simulink model "test_loopback_mux"  (Simulink 7.0)
settings: Solver=ode45  StartTime=0.0  StopTime=4000  RelTol=1e-3
libraries: xbsIndex_r4 x498, xps_library x21, xbsReplacements_r4 x18, casper_library x15
(part 1 of 3)
settings Model: Creator=dsp  LastModifiedBy=dsp
settings DebuggingCC: SaveWithParameterizedLinksMsg=none  SignalResolutionControl=TryResolveAllWithWarning  MultiTaskDSMMsg=warning  MultiTaskCondExecSysMsg=none  StrictBusMsg=None
settings RTWCC: IncludeERTFirstTime=on
settings GRTTargetCC: TargetFcnLib=ansi_tfl_tmw.mat

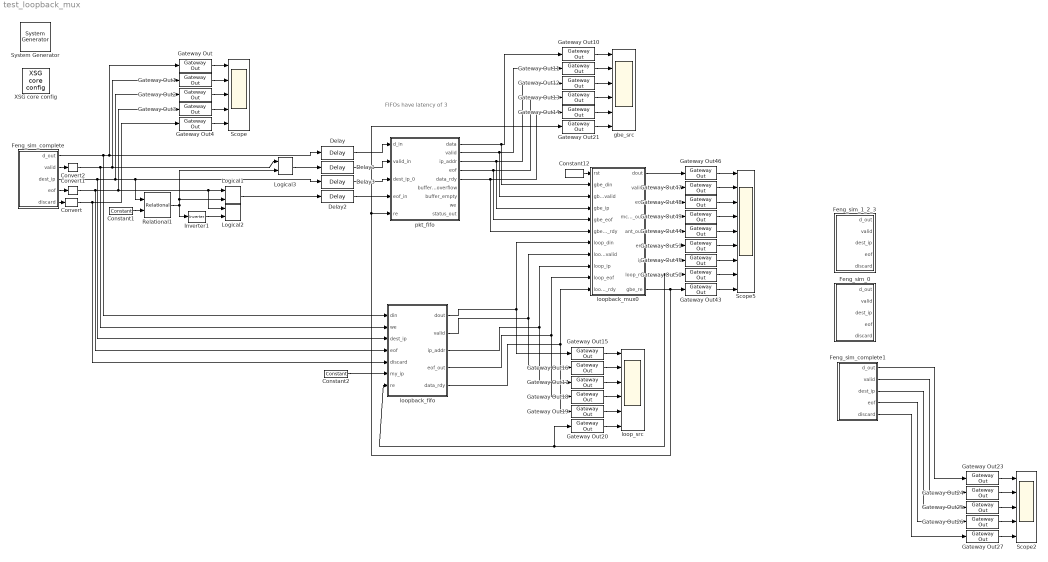
== system test_loopback_mux ==
  note: FIFOs have latency of 3
  " System Generator" : xbsIndex_r4/ System Generator  Tag=genX  SystemSampleTime=-1  xilinxfamily=Virtex2P  part=xc2vp70  speed=-7  package=ff1704  synthesis_tool=XST  clock_wrapper=Clock Enables  directory=./b_2x_8a_r308d/sysgen  testbench=off  simulink_period=1  sysclk_period=4.878  dcm_input_clock_period=100  incr_netlist=off  trim_vbits=Everywhere in SubSystem  dbl_ovrd=According to Block Masks  core_generation=According to Block Masks  run_coregen=off  deprecated_control=off  eval_field=0  block_type=sysgen
      settings: block_version=10.1.3
  Constant1 : xbsIndex_r4/Constant  arith_type=Unsigned  const=0  n_bits=1  bin_pt=0  explicit_period=on  period=1  equ=P=C  opselect=C  inp2=PCIN>>17  opr=+  inp1=P  carry=CIN  dbl_ovrd=off  block_type=constant
  Constant12 : xbsIndex_r4/Constant  arith_type=Boolean  const=0  n_bits=1  bin_pt=0  explicit_period=on  period=1  equ=P=C  opselect=C  inp2=PCIN>>17  opr=+  inp1=P  carry=CIN  dbl_ovrd=off  block_type=constant
  Constant2 : xbsIndex_r4/Constant  arith_type=Unsigned  const=0  n_bits=32  bin_pt=0  explicit_period=on  period=1  equ=P=C  opselect=C  inp2=PCIN>>17  opr=+  inp1=P  carry=CIN  dbl_ovrd=off  block_type=constant
  Convert : xbsIndex_r4/Convert  arith_type=Boolean  n_bits=8  bin_pt=6  quantization=Truncate  overflow=Wrap  latency=0  dbl_ovrd=off  pipeline=off  block_type=convert
      settings: xl_area=[0, 0, 0, 0, 0, 0, 0]  block_version=10.1.3
  Convert1 : xbsIndex_r4/Convert  arith_type=Boolean  n_bits=8  bin_pt=6  quantization=Truncate  overflow=Wrap  latency=0  dbl_ovrd=off  pipeline=off  block_type=convert
      settings: xl_area=[0, 0, 0, 0, 0, 0, 0]  block_version=10.1.3
  Convert2 : xbsIndex_r4/Convert  arith_type=Boolean  n_bits=8  bin_pt=6  quantization=Truncate  overflow=Wrap  latency=0  dbl_ovrd=off  pipeline=off  block_type=convert
      settings: xl_area=[0, 0, 0, 0, 0, 0, 0]  block_version=10.1.3
  Delay{,1..3} (4 alike) : xbsIndex_r4/Delay  en=off  latency=220  dbl_ovrd=off  reg_retiming=off  block_type=delay
      settings: xl_area=[0, 0, 0, 0, 0, 0, 0]
  Feng_sim_0 : Subsystem
  Feng_sim_1_2_3 : Subsystem
  Feng_sim_complete : Subsystem
  Feng_sim_complete1 : Subsystem
  Gateway Out{,1..4,10..21,23..27,43..51} (31 alike) : xbsIndex_r4/Gateway Out  hdl_port=on  timing_constraint=None  locs_specified=off  LOCs={}  block_type=gatewayout
      settings: infoedit="Gateway out block.  Converts Xilinx fixed point inputs into ouputs of type Simulink integer, double, or fixed point.<P><P>Hardware notes:  In hardware these blocks become top level output ports or are discarded, depending on how they are configured."  xl_area=[0, 0, 0, 0, 0, 0, 0]  block_version=10.1.3
  Inverter1 : xbsIndex_r4/Inverter  en=off  latency=0  dbl_ovrd=off  block_type=inv
      settings: xl_area=[0, 0, 0, 0, 0, 0, 0]
  Logical1 : xbsIndex_r4/Logical  logical_function=AND  inputs=2  en=off  latency=0  precision=Full  arith_type=Unsigned  n_bits=8  bin_pt=2  align_bp=on  dbl_ovrd=off  block_type=logical
      settings: xl_area=[0, 0, 0, 0, 0, 0, 0]
  Logical2 : xbsIndex_r4/Logical  logical_function=AND  inputs=2  en=off  latency=0  precision=Full  arith_type=Unsigned  n_bits=8  bin_pt=2  align_bp=on  dbl_ovrd=off  block_type=logical
      settings: xl_area=[0, 0, 0, 0, 0, 0, 0]
  Logical3 : xbsIndex_r4/Logical  logical_function=AND  inputs=2  en=off  latency=0  precision=Full  arith_type=Unsigned  n_bits=8  bin_pt=2  align_bp=on  dbl_ovrd=off  block_type=logical
      settings: xl_area=[0, 0, 0, 0, 0, 0, 0]
  Relational1 : xbsIndex_r4/Relational  mode=a!=b  en=off  latency=0  dbl_ovrd=off  block_type=relational
      settings: xl_area=[0, 0, 0, 0, 0, 0, 0]  block_version=10.1.3
  Scope : Scope  NumInputPorts=5
      settings: TimeRange=10000  YMin=0~0~0~0~-1  YMax=5000~1~3~1~1
  Scope2 : Scope  NumInputPorts=5
      settings: TimeRange=10000  YMin=0~0~0~0~-1  YMax=5000~1~3~1~1  SaveName=ScopeData12
  Scope5 : Scope  NumInputPorts=9
      settings: YMin=1100~0~0~-1~0.95~-5~-5~-5~-5  YMax=1200~1~1~1~1.05~5~5~5~5  SaveName=ScopeData17
  XSG core config : xps_library/XSG core config  Tag=xps:xsg  SystemSampleTime=-1  hw_sys=BEE2_usr  ibob_linux=off  clk_src=sys_clk  iBOB_clk_src=sys_clk  BEE2_ctrl_clk_src=sys_clk  BEE2_usr_clk_src=sys_clk  ROACH_clk_src=sys_clk  CORR_clk_src=sys_clk  gpio_clk_io_group=iBOB:sma  gpio_clk_bit_index=0  clk_rate=100  sample_period=1  synthesis_tool=XST  mpc_type=powerpc405
  gbe_src : Scope  NumInputPorts=6
      settings: YMin=95.95~0.95~1.9~-1~-1~-1  YMax=106.05~1.05~2.1~1~1~1  SaveName=ScopeData4
  loop_src : Scope  NumInputPorts=6
      settings: YMin=95.95~0.95~1.9~-1~-1~-1  YMax=106.05~1.05~2.1~1~1~1
  loopback_fifo : Subsystem
  loopback_mux0 : Subsystem  mask{timeout_bits=12, payload_len=50, fifo_latency=3}
      mask prompts: timeout_bits "Timeout (clock cycles, 2^?)"; payload_len "Expected payload length (in 64bit words)"; fifo_latency "Input pkt_fifo latencies"
      mask init:
      | payload_bits = ceil(log2(payload_len));
      | fmtstr = sprintf('Payload Len: %i\nFIFO latencies: %i.', payload_len,fifo_latency);
      | set_param(gcb, 'AttributesFormatString', fmtstr);
      settings: AttributesFormatString=|
      | Payload Len: 50
      | FIFO latencies: 3.
  pkt_fifo : Subsystem
      settings: AttributesFormatString=|
      | Max 1024 data words.
      | Max 32 pkts.
  wires:
  Feng_sim_complete/1(d_out) -> Gateway Out/1, Delay/1, loopback_fifo/1(din)
  Feng_sim_complete/2(valid) -> Convert2/1
  Feng_sim_complete/4(eof) -> Convert1/1
  Feng_sim_complete/3(dest_ip) -> Gateway Out2/1, Relational1/1, Delay3/1, loopback_fifo/3(dest_ip)
  Feng_sim_complete/5(discard) -> Convert/1
  Gateway Out/1 -> Scope/1
  Gateway Out1/1 -> Scope/2
  Gateway Out2/1 -> Scope/3
  Gateway Out3/1 -> Scope/4
  Gateway Out4/1 -> Scope/5
  Inverter1/1 -> Logical2/2
  Relational1/1 -> Inverter1/1, Logical1/2, Logical3/2
  Logical1/1 -> Delay2/1
  Constant1/1 -> Relational1/2
  Gateway Out10/1 -> gbe_src/1
  Gateway Out11/1 -> gbe_src/2
  Gateway Out12/1 -> gbe_src/3
  Gateway Out13/1 -> gbe_src/4
  Gateway Out14/1 -> gbe_src/5
  Gateway Out21/1 -> gbe_src/6
  Feng_sim_complete1/1(d_out) -> Gateway Out23/1
  Feng_sim_complete1/2(valid) -> Gateway Out24/1
  Feng_sim_complete1/3(dest_ip) -> Gateway Out25/1
  Feng_sim_complete1/4(eof) -> Gateway Out26/1
  Feng_sim_complete1/5(discard) -> Gateway Out27/1
  Gateway Out23/1 -> Scope2/1
  Gateway Out24/1 -> Scope2/2
  Gateway Out25/1 -> Scope2/3
  Gateway Out26/1 -> Scope2/4
  Gateway Out27/1 -> Scope2/5
  Gateway Out46/1 -> Scope5/1
  Gateway Out47/1 -> Scope5/2
  Gateway Out48/1 -> Scope5/3
  Gateway Out49/1 -> Scope5/4
  Gateway Out44/1 -> Scope5/5
  pkt_fifo/1(data) -> Gateway Out10/1, loopback_mux0/2(gbe_din)
  pkt_fifo/2(valid) -> Gateway Out11/1, loopback_mux0/3(gbe_valid)
  pkt_fifo/3(ip_addr) -> Gateway Out12/1, loopback_mux0/4(gbe_ip)
  Gateway Out15/1 -> loop_src/1
  Gateway Out16/1 -> loop_src/2
  Gateway Out17/1 -> loop_src/3
  Gateway Out18/1 -> loop_src/4
  Gateway Out19/1 -> loop_src/5
  Gateway Out20/1 -> loop_src/6
  Gateway Out51/1 -> Scope5/6
  Gateway Out45/1 -> Scope5/7
  Gateway Out50/1 -> Scope5/8
  Gateway Out43/1 -> Scope5/9
  loopback_mux0/1(dout) -> Gateway Out46/1
  loopback_mux0/2(valid) -> Gateway Out47/1
  loopback_mux0/3(eof) -> Gateway Out48/1
  loopback_mux0/4(mcnt_out) -> Gateway Out49/1
  loopback_mux0/5(ant_out) -> Gateway Out44/1
  loopback_mux0/6(err) -> Gateway Out51/1
  loopback_mux0/7(ip) -> Gateway Out45/1
  loopback_mux0/8(loop_re) -> Gateway Out50/1, Gateway Out20/1, loopback_fifo/7(re)
  loopback_mux0/9(gbe_re) -> Gateway Out43/1, pkt_fifo/5(re), Gateway Out21/1
  Logical3/1 -> Delay1/1
  Delay/1 -> pkt_fifo/1(d_in)
  Delay1/1 -> pkt_fifo/2(valid_in)
  Delay3/1 -> pkt_fifo/3(dest_ip_0)
  Delay2/1 -> pkt_fifo/4(eof_in)
  pkt_fifo/4(eof) -> Gateway Out13/1, loopback_mux0/5(gbe_eof)
  Constant12/1 -> loopback_mux0/1(rst)
  loopback_fifo/1(dout) -> loopback_mux0/7(loop_din), Gateway Out15/1
  loopback_fifo/2(valid) -> loopback_mux0/8(loop_valid), Gateway Out16/1
  loopback_fifo/3(ip_addr) -> loopback_mux0/9(loop_ip), Gateway Out17/1
  pkt_fifo/5(data_rdy) -> Gateway Out14/1, loopback_mux0/6(gbe_data_rdy)
  loopback_fifo/5(data_rdy) -> loopback_mux0/11(loop_data_rdy), Gateway Out19/1
  Convert/1 -> Gateway Out4/1, loopback_fifo/5(discard)
  Convert1/1 -> Gateway Out3/1, Logical1/1, Logical2/1, loopback_fifo/4(eof)
  Convert2/1 -> Gateway Out1/1, Logical3/1, loopback_fifo/2(we)
  Constant2/1 -> loopback_fifo/6(my_ip)
  loopback_fifo/4(eof_out) -> loopback_mux0/10(loop_eof), Gateway Out18/1

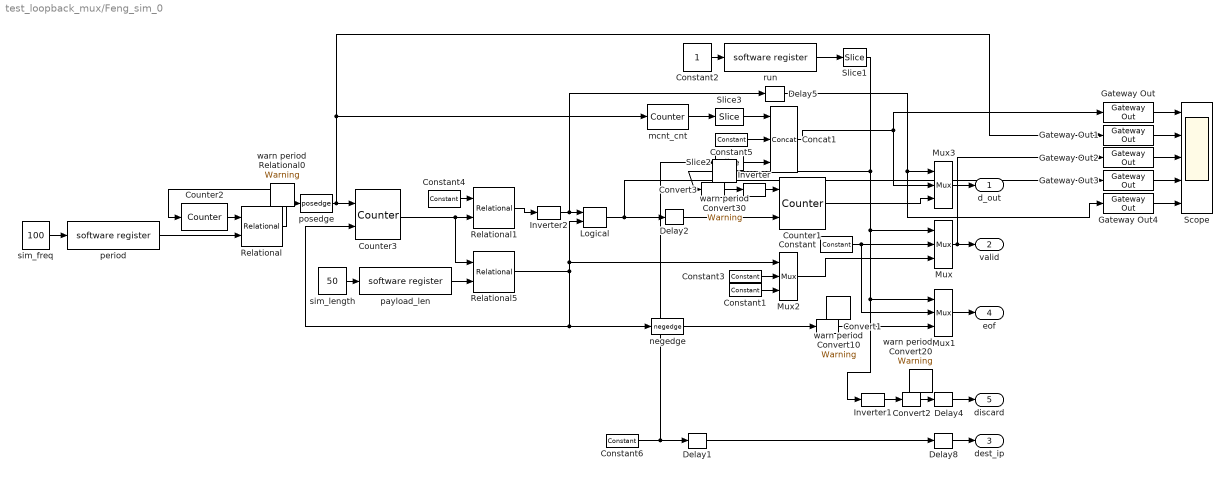
== system test_loopback_mux/Feng_sim_0 ==
  Concat1 : xbsIndex_r4/Concat  num_inputs=3  dbl_ovrd=off  block_type=concat
      settings: block_version=10.1.3
  Constant : xbsIndex_r4/Constant  arith_type=Boolean  const=0  n_bits=1  bin_pt=0  explicit_period=on  period=1  equ=P=C  opselect=C  inp2=PCIN>>17  opr=+  inp1=P  carry=CIN  dbl_ovrd=off  block_type=constant
  Constant1 : xbsIndex_r4/Constant  arith_type=Boolean  const=1  n_bits=1  bin_pt=0  explicit_period=off  period=1  equ=P=C  opselect=C  inp2=PCIN>>17  opr=+  inp1=P  carry=CIN  dbl_ovrd=off  block_type=constant
  Constant2 : Constant  OutDataType=sfix(16)  OutScaling=2^0
  Constant3 : xbsIndex_r4/Constant  arith_type=Boolean  const=0  n_bits=1  bin_pt=0  explicit_period=off  period=1  equ=P=C  opselect=C  inp2=PCIN>>17  opr=+  inp1=P  carry=CIN  dbl_ovrd=off  block_type=constant
  Constant4 : xbsIndex_r4/Constant  arith_type=Unsigned  const=0  n_bits=32  bin_pt=0  explicit_period=on  period=1  equ=P=C  opselect=C  inp2=PCIN>>17  opr=+  inp1=P  carry=CIN  dbl_ovrd=off  block_type=constant
  Constant5 : xbsIndex_r4/Constant  arith_type=Unsigned  const=0  n_bits=16-2  bin_pt=0  explicit_period=on  period=1  equ=P=C  opselect=C  inp2=PCIN>>17  opr=+  inp1=P  carry=CIN  dbl_ovrd=off  block_type=constant
  Constant6 : xbsIndex_r4/Constant  arith_type=Unsigned  const=0  n_bits=32  bin_pt=0  explicit_period=on  period=1  equ=P=C  opselect=C  inp2=PCIN>>17  opr=+  inp1=P  carry=CIN  dbl_ovrd=off  block_type=constant
  Convert1 : xbsIndex_r4/Convert  arith_type=Boolean  n_bits=8  bin_pt=6  quantization=Truncate  overflow=Wrap  latency=0  dbl_ovrd=off  pipeline=off  block_type=convert
      settings: xl_area=[0, 0, 0, 0, 0, 0, 0]  block_version=10.1.3
  Convert2 : xbsIndex_r4/Convert  arith_type=Boolean  n_bits=8  bin_pt=6  quantization=Truncate  overflow=Wrap  latency=0  dbl_ovrd=off  pipeline=off  block_type=convert
      settings: xl_area=[0, 0, 0, 0, 0, 0, 0]  block_version=10.1.3
  Convert3 : xbsIndex_r4/Convert  arith_type=Boolean  n_bits=8  bin_pt=6  quantization=Truncate  overflow=Wrap  latency=0  dbl_ovrd=off  pipeline=off  block_type=convert
      settings: xl_area=[0, 0, 0, 0, 0, 0, 0]  block_version=10.1.3
  Counter1 : xbsIndex_r4/Counter  cnt_type=Free Running  cnt_to=Inf  operation=Up  start_count=0  cnt_by_val=1  arith_type=Unsigned  n_bits=64  bin_pt=0  load_pin=off  rst=on  en=on  explicit_period=off  period=1  dbl_ovrd=off  use_behavioral_HDL=off  use_rpm=off  implementation=Fabric  block_type=counter
      settings: xl_area=[0, 0, 0, 0, 0, 0, 0]
  Counter2 : xbsIndex_r4/Counter  cnt_type=Free Running  cnt_to=Inf  operation=Up  start_count=1  cnt_by_val=1  arith_type=Unsigned  n_bits=32  bin_pt=0  load_pin=off  rst=on  en=off  explicit_period=on  period=1  dbl_ovrd=off  use_behavioral_HDL=off  use_rpm=on  implementation=Fabric  block_type=counter
      settings: xl_area=[0, 0, 0, 0, 0, 0, 0]
  Counter3 : xbsIndex_r4/Counter  cnt_type=Free Running  cnt_to=1023  operation=Up  start_count=0  cnt_by_val=1  arith_type=Unsigned  n_bits=32  bin_pt=0  load_pin=off  rst=on  en=on  explicit_period=on  period=1  dbl_ovrd=off  use_behavioral_HDL=off  use_rpm=on  implementation=Fabric  block_type=counter
      settings: xl_area=[0, 0, 0, 0, 0, 0, 0]
  Delay{1..2,4..5,8} (5 alike) : xbsIndex_r4/Delay  en=off  latency=1  dbl_ovrd=off  reg_retiming=on  block_type=delay
      settings: xl_area=[0, 0, 0, 0, 0, 0, 0]
  Gateway Out{,1..4} (5 alike) : xbsIndex_r4/Gateway Out  hdl_port=on  timing_constraint=None  locs_specified=off  LOCs={}  block_type=gatewayout
      settings: infoedit="Gateway out block.  Converts Xilinx fixed point inputs into ouputs of type Simulink integer, double, or fixed point.<P><P>Hardware notes:  In hardware these blocks become top level output ports or are discarded, depending on how they are configured."  xl_area=[0, 0, 0, 0, 0, 0, 0]  block_version=10.1.3
  Inverter : xbsIndex_r4/Inverter  en=off  latency=0  dbl_ovrd=off  block_type=inv
      settings: xl_area=[0, 0, 0, 0, 0, 0, 0]
  Inverter1 : xbsIndex_r4/Inverter  en=off  latency=0  dbl_ovrd=off  block_type=inv
      settings: xl_area=[0, 0, 0, 0, 0, 0, 0]
  Inverter2 : xbsIndex_r4/Inverter  en=off  latency=0  dbl_ovrd=off  block_type=inv
      settings: xl_area=[0, 0, 0, 0, 0, 0, 0]
  Logical : xbsIndex_r4/Logical  logical_function=AND  inputs=2  en=off  latency=0  precision=Full  arith_type=Unsigned  n_bits=8  bin_pt=2  align_bp=on  dbl_ovrd=off  block_type=logical
      settings: xl_area=[0, 0, 0, 0, 0, 0, 0]
  Mux{,1..3} (4 alike) : xbsIndex_r4/Mux  inputs=2  en=off  latency=1  precision=Full  arith_type="Signed  (2's comp)"  n_bits=8  bin_pt=2  quantization=Truncate  overflow=Wrap  dbl_ovrd=off  block_type=mux
      settings: xl_area=[0, 0, 0, 0, 0, 0, 0]
  Relational : xbsIndex_r4/Relational  mode=a>=b  en=off  latency=0  dbl_ovrd=off  block_type=relational
      settings: xl_area=[0, 0, 0, 0, 0, 0, 0]  block_version=10.1.3
  Relational1 : xbsIndex_r4/Relational  mode=a=b  en=off  latency=0  dbl_ovrd=off  block_type=relational
      settings: xl_area=[0, 0, 0, 0, 0, 0, 0]  block_version=10.1.3
  Relational5 : xbsIndex_r4/Relational  mode=a<=b  en=off  latency=0  dbl_ovrd=off  block_type=relational
      settings: xl_area=[0, 0, 0, 0, 0, 0, 0]  block_version=10.1.3
  Scope : Scope  NumInputPorts=5
      settings: TimeRange=4000  YMin=130000~0~0~0~0  YMax=200000~1~1~1~1  SaveName=ScopeData11
  Slice1 : xbsIndex_r4/Slice  nbits=1  boolean_output=off  mode=Lower Bit Location + Width  bit1=1  base1=MSB of Input  bit0=0  base0=LSB of Input  dbl_ovrd=off  block_type=slice
      settings: infoedit="Extracts a given range of bits from each input sample and presents it at the output.  The output type is ordinarily unsigned with binary point at zero, but can be Boolean when the slice is one bit wide.<P><P>Hardware notes: In hardware this block costs nothing."  block_version=10.1.3
  Slice2 : xbsIndex_r4/Slice  nbits=2  boolean_output=off  mode=Lower Bit Location + Width  bit1=1  base1=MSB of Input  bit0=0  base0=LSB of Input  dbl_ovrd=off  block_type=slice
      settings: infoedit="Extracts a given range of bits from each input sample and presents it at the output.  The output type is ordinarily unsigned with binary point at zero, but can be Boolean when the slice is one bit wide.<P><P>Hardware notes: In hardware this block costs nothing."  block_version=10.1.3
  Slice3 : xbsIndex_r4/Slice  nbits=48  boolean_output=off  mode=Lower Bit Location + Width  bit1=1  base1=MSB of Input  bit0=2  base0=LSB of Input  dbl_ovrd=off  block_type=slice
      settings: infoedit="Extracts a given range of bits from each input sample and presents it at the output.  The output type is ordinarily unsigned with binary point at zero, but can be Boolean when the slice is one bit wide.<P><P>Hardware notes: In hardware this block costs nothing."  block_version=10.1.3
  mcnt_cnt : xbsIndex_r4/Counter  cnt_type=Free Running  cnt_to=Inf  operation=Up  start_count=0  cnt_by_val=1  arith_type=Unsigned  n_bits=64  bin_pt=0  load_pin=off  rst=off  en=on  explicit_period=off  period=1  dbl_ovrd=off  use_behavioral_HDL=off  use_rpm=off  implementation=Fabric  block_type=counter
      settings: xl_area=[0, 0, 0, 0, 0, 0, 0]
  negedge : casper_library/Misc/negedge  Tag=Rising Edge Detector  SystemSampleTime=-1
  payload_len : xps_library/software register  Tag=xps:sw_reg  SystemSampleTime=-1  io_dir=From Processor  arith_type=Unsigned  bitwidth=32  bin_pt=0  sample_period=1  gw_name=test_loopback_mux_Feng_sim_0_payload_len_user_data_out
      link override test_loopback_mux_Feng_sim_0_payload_len_user_data_out: arith_type=Unsigned  n_bits=32  bin_pt=0  period=1
  period : xps_library/software register  Tag=xps:sw_reg  SystemSampleTime=-1  io_dir=From Processor  arith_type=Unsigned  bitwidth=32  bin_pt=0  sample_period=1  gw_name=test_loopback_mux_Feng_sim_0_period_user_data_out
      link override test_loopback_mux_Feng_sim_0_period_user_data_out: arith_type=Unsigned  n_bits=32  bin_pt=0  period=1
  posedge : casper_library/Misc/pulse_ext/posedge  Tag=Rising Edge Detector  SystemSampleTime=-1
  run : xps_library/software register  Tag=xps:sw_reg  SystemSampleTime=-1  io_dir=From Processor  arith_type=Unsigned  bitwidth=32  bin_pt=0  sample_period=1  gw_name=test_loopback_mux_Feng_sim_0_run_user_data_out
      link override test_loopback_mux_Feng_sim_0_run_user_data_out: arith_type=Unsigned  n_bits=32  bin_pt=0  period=1
  sim_freq : Constant  Value=100  OutDataType=sfix(16)  OutScaling=2^0
  sim_length : Constant  Value=50  OutDataType=sfix(16)  OutScaling=2^0
  warn period Convert10 : xbsReplacements_r4/Warning  SystemSampleTime=-1  period=1
  warn period Convert20 : xbsReplacements_r4/Warning  SystemSampleTime=-1  period=1
  warn period Convert30 : xbsReplacements_r4/Warning  SystemSampleTime=-1  period=1
  warn period Relational0 : xbsReplacements_r4/Warning  SystemSampleTime=-1  period=1
  d_out : Outport  OutDataType=sfix(16)  OutScaling=2^0
  valid : Outport  Port=2  OutDataType=sfix(16)  OutScaling=2^0
  dest_ip : Outport  Port=3  OutDataType=sfix(16)  OutScaling=2^0
  eof : Outport  Port=4  OutDataType=sfix(16)  OutScaling=2^0
  discard : Outport  Port=5  OutDataType=sfix(16)  OutScaling=2^0
  wires:
  Delay1/1 -> Delay8/1
  Slice2/1 -> Concat1/3
  Slice3/1 -> Concat1/1
  Logical/1 -> Gateway Out3/1, Delay2/1
  Gateway Out4/1 -> Scope/5
  Gateway Out3/1 -> Scope/4
  Gateway Out2/1 -> Scope/3
  Gateway Out1/1 -> Scope/2
  Gateway Out/1 -> Scope/1
  Delay5/1 -> Gateway Out4/1, Mux3/1
  Concat1/1 -> Gateway Out/1, Mux3/2
  Constant5/1 -> Concat1/2
  mcnt_cnt/1 -> Slice3/1
  Inverter2/1 -> Logical/1, Delay5/1
  Relational1/1 -> Inverter2/1
  Constant4/1 -> Relational1/1
  Constant6/1 -> Slice2/1, Delay1/1
  Convert2/1 -> Delay4/1
  Inverter1/1 -> Convert2/1
  Constant1/1 -> Mux2/3
  Constant3/1 -> Mux2/2
  Convert3/1 -> Inverter/1
  Delay2/1 -> Counter1/2
  Inverter/1 -> Counter1/1
  Mux2/1 -> Mux/3
  Delay4/1 -> discard/1
  Slice1/1 -> Convert3/1, Inverter1/1, Mux1/1, Mux/1
  Constant2/1 -> run/1
  run/1 -> Slice1/1
  Delay8/1 -> dest_ip/1
  Mux3/1 -> d_out/1
  Convert1/1 -> Mux1/3
  Mux1/1 -> eof/1
  Constant/1 -> Mux1/2, Mux/2
  Mux/1 -> Gateway Out2/1, valid/1
  payload_len/1 -> Relational5/2
  sim_length/1 -> payload_len/1
  posedge/1 -> Gateway Out1/1, mcnt_cnt/1, Counter3/1
  Counter3/1 -> Relational1/2, Relational5/1
  Relational5/1 -> Counter3/2, negedge/1, Mux2/1, Logical/2
  sim_freq/1 -> period/1
  period/1 -> Relational/2
  negedge/1 -> Convert1/1
  Counter1/1 -> Mux3/3
  Relational/1 -> Counter2/1, posedge/1
  Counter2/1 -> Relational/1

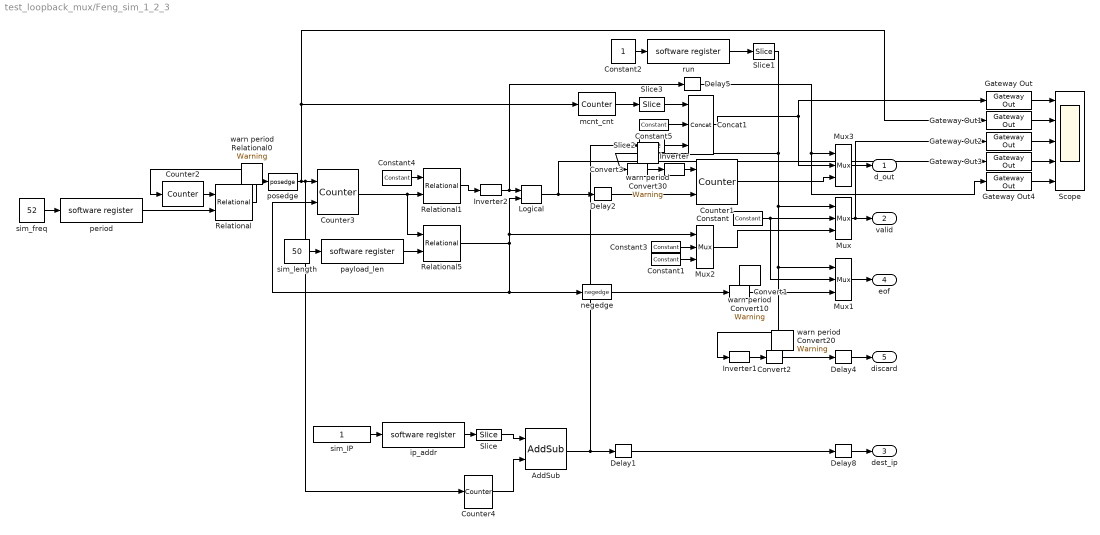
== system test_loopback_mux/Feng_sim_1_2_3 ==
  AddSub : xbsIndex_r4/AddSub  mode=Addition  use_carryin=off  use_carryout=off  en=off  latency=0  precision=Full  arith_type=Unsigned  n_bits=8  bin_pt=2  quantization=Truncate  overflow=Wrap  dbl_ovrd=off  use_behavioral_HDL=on  pipelined=off  use_rpm=on  hw_selection=Fabric  block_type=addsub
      settings: xl_area=[0, 0, 0, 0, 0, 0, 0]  block_version=10.1.3
  Concat1 : xbsIndex_r4/Concat  num_inputs=3  dbl_ovrd=off  block_type=concat
      settings: block_version=10.1.3
  Constant : xbsIndex_r4/Constant  arith_type=Boolean  const=0  n_bits=1  bin_pt=0  explicit_period=on  period=1  equ=P=C  opselect=C  inp2=PCIN>>17  opr=+  inp1=P  carry=CIN  dbl_ovrd=off  block_type=constant
  Constant1 : xbsIndex_r4/Constant  arith_type=Boolean  const=1  n_bits=1  bin_pt=0  explicit_period=off  period=1  equ=P=C  opselect=C  inp2=PCIN>>17  opr=+  inp1=P  carry=CIN  dbl_ovrd=off  block_type=constant
  Constant2 : Constant  OutDataType=sfix(16)  OutScaling=2^0
  Constant3 : xbsIndex_r4/Constant  arith_type=Boolean  const=0  n_bits=1  bin_pt=0  explicit_period=off  period=1  equ=P=C  opselect=C  inp2=PCIN>>17  opr=+  inp1=P  carry=CIN  dbl_ovrd=off  block_type=constant
  Constant4 : xbsIndex_r4/Constant  arith_type=Unsigned  const=0  n_bits=32  bin_pt=0  explicit_period=on  period=1  equ=P=C  opselect=C  inp2=PCIN>>17  opr=+  inp1=P  carry=CIN  dbl_ovrd=off  block_type=constant
  Constant5 : xbsIndex_r4/Constant  arith_type=Unsigned  const=0  n_bits=16-2  bin_pt=0  explicit_period=on  period=1  equ=P=C  opselect=C  inp2=PCIN>>17  opr=+  inp1=P  carry=CIN  dbl_ovrd=off  block_type=constant
  Convert1 : xbsIndex_r4/Convert  arith_type=Boolean  n_bits=8  bin_pt=6  quantization=Truncate  overflow=Wrap  latency=0  dbl_ovrd=off  pipeline=off  block_type=convert
      settings: xl_area=[0, 0, 0, 0, 0, 0, 0]  block_version=10.1.3
  Convert2 : xbsIndex_r4/Convert  arith_type=Boolean  n_bits=8  bin_pt=6  quantization=Truncate  overflow=Wrap  latency=0  dbl_ovrd=off  pipeline=off  block_type=convert
      settings: xl_area=[0, 0, 0, 0, 0, 0, 0]  block_version=10.1.3
  Convert3 : xbsIndex_r4/Convert  arith_type=Boolean  n_bits=8  bin_pt=6  quantization=Truncate  overflow=Wrap  latency=0  dbl_ovrd=off  pipeline=off  block_type=convert
      settings: xl_area=[0, 0, 0, 0, 0, 0, 0]  block_version=10.1.3
  Counter1 : xbsIndex_r4/Counter  cnt_type=Free Running  cnt_to=Inf  operation=Up  start_count=0  cnt_by_val=1  arith_type=Unsigned  n_bits=64  bin_pt=0  load_pin=off  rst=on  en=on  explicit_period=off  period=1  dbl_ovrd=off  use_behavioral_HDL=off  use_rpm=off  implementation=Fabric  block_type=counter
      settings: xl_area=[0, 0, 0, 0, 0, 0, 0]
  Counter2 : xbsIndex_r4/Counter  cnt_type=Free Running  cnt_to=Inf  operation=Up  start_count=1  cnt_by_val=1  arith_type=Unsigned  n_bits=32  bin_pt=0  load_pin=off  rst=on  en=off  explicit_period=on  period=1  dbl_ovrd=off  use_behavioral_HDL=off  use_rpm=on  implementation=Fabric  block_type=counter
      settings: xl_area=[0, 0, 0, 0, 0, 0, 0]
  Counter3 : xbsIndex_r4/Counter  cnt_type=Free Running  cnt_to=1023  operation=Up  start_count=0  cnt_by_val=1  arith_type=Unsigned  n_bits=32  bin_pt=0  load_pin=off  rst=on  en=on  explicit_period=on  period=1  dbl_ovrd=off  use_behavioral_HDL=off  use_rpm=on  implementation=Fabric  block_type=counter
      settings: xl_area=[0, 0, 0, 0, 0, 0, 0]
  Counter4 : xbsIndex_r4/Counter  cnt_type=Count Limited  cnt_to=2  operation=Up  start_count=0  cnt_by_val=1  arith_type=Unsigned  n_bits=2  bin_pt=0  load_pin=off  rst=off  en=on  explicit_period=on  period=1  dbl_ovrd=off  use_behavioral_HDL=off  use_rpm=on  implementation=Fabric  block_type=counter
      settings: xl_area=[0, 0, 0, 0, 0, 0, 0]
  Delay{1..2,4..5,8} (5 alike) : xbsIndex_r4/Delay  en=off  latency=1  dbl_ovrd=off  reg_retiming=on  block_type=delay
      settings: xl_area=[0, 0, 0, 0, 0, 0, 0]
  Gateway Out{,1..4} (5 alike) : xbsIndex_r4/Gateway Out  hdl_port=on  timing_constraint=None  locs_specified=off  LOCs={}  block_type=gatewayout
      settings: infoedit="Gateway out block.  Converts Xilinx fixed point inputs into ouputs of type Simulink integer, double, or fixed point.<P><P>Hardware notes:  In hardware these blocks become top level output ports or are discarded, depending on how they are configured."  xl_area=[0, 0, 0, 0, 0, 0, 0]  block_version=10.1.3
  Inverter : xbsIndex_r4/Inverter  en=off  latency=0  dbl_ovrd=off  block_type=inv
      settings: xl_area=[0, 0, 0, 0, 0, 0, 0]
  Inverter1 : xbsIndex_r4/Inverter  en=off  latency=0  dbl_ovrd=off  block_type=inv
      settings: xl_area=[0, 0, 0, 0, 0, 0, 0]
  Inverter2 : xbsIndex_r4/Inverter  en=off  latency=0  dbl_ovrd=off  block_type=inv
      settings: xl_area=[0, 0, 0, 0, 0, 0, 0]
  Logical : xbsIndex_r4/Logical  logical_function=AND  inputs=2  en=off  latency=0  precision=Full  arith_type=Unsigned  n_bits=8  bin_pt=2  align_bp=on  dbl_ovrd=off  block_type=logical
      settings: xl_area=[0, 0, 0, 0, 0, 0, 0]
  Mux{,1..3} (4 alike) : xbsIndex_r4/Mux  inputs=2  en=off  latency=1  precision=Full  arith_type="Signed  (2's comp)"  n_bits=8  bin_pt=2  quantization=Truncate  overflow=Wrap  dbl_ovrd=off  block_type=mux
      settings: xl_area=[0, 0, 0, 0, 0, 0, 0]
  Relational : xbsIndex_r4/Relational  mode=a>=b  en=off  latency=0  dbl_ovrd=off  block_type=relational
      settings: xl_area=[0, 0, 0, 0, 0, 0, 0]  block_version=10.1.3
  Relational1 : xbsIndex_r4/Relational  mode=a=b  en=off  latency=0  dbl_ovrd=off  block_type=relational
      settings: xl_area=[0, 0, 0, 0, 0, 0, 0]  block_version=10.1.3
  Relational5 : xbsIndex_r4/Relational  mode=a<=b  en=off  latency=0  dbl_ovrd=off  block_type=relational
      settings: xl_area=[0, 0, 0, 0, 0, 0, 0]  block_version=10.1.3
  Scope : Scope  NumInputPorts=5
      settings: TimeRange=4000  YMin=130000~0~0~0~0  YMax=200000~1~1~1~1  SaveName=ScopeData11
  Slice : xbsIndex_r4/Slice  nbits=31  boolean_output=off  mode=Lower Bit Location + Width  bit1=0  base1=MSB of Input  bit0=0  base0=LSB of Input  dbl_ovrd=off  block_type=slice
      settings: infoedit="Extracts a given range of bits from each input sample and presents it at the output.  The output type is ordinarily unsigned with binary point at zero, but can be Boolean when the slice is one bit wide.<P><P>Hardware notes: In hardware this block costs nothing."  block_version=10.1.3
  Slice1 : xbsIndex_r4/Slice  nbits=1  boolean_output=off  mode=Lower Bit Location + Width  bit1=1  base1=MSB of Input  bit0=0  base0=LSB of Input  dbl_ovrd=off  block_type=slice
      settings: infoedit="Extracts a given range of bits from each input sample and presents it at the output.  The output type is ordinarily unsigned with binary point at zero, but can be Boolean when the slice is one bit wide.<P><P>Hardware notes: In hardware this block costs nothing."  block_version=10.1.3
  Slice2 : xbsIndex_r4/Slice  nbits=2  boolean_output=off  mode=Lower Bit Location + Width  bit1=1  base1=MSB of Input  bit0=0  base0=LSB of Input  dbl_ovrd=off  block_type=slice
      settings: infoedit="Extracts a given range of bits from each input sample and presents it at the output.  The output type is ordinarily unsigned with binary point at zero, but can be Boolean when the slice is one bit wide.<P><P>Hardware notes: In hardware this block costs nothing."  block_version=10.1.3
  Slice3 : xbsIndex_r4/Slice  nbits=48  boolean_output=off  mode=Lower Bit Location + Width  bit1=1  base1=MSB of Input  bit0=3  base0=LSB of Input  dbl_ovrd=off  block_type=slice
      settings: infoedit="Extracts a given range of bits from each input sample and presents it at the output.  The output type is ordinarily unsigned with binary point at zero, but can be Boolean when the slice is one bit wide.<P><P>Hardware notes: In hardware this block costs nothing."  block_version=10.1.3
  ip_addr : xps_library/software register  Tag=xps:sw_reg  SystemSampleTime=-1  io_dir=From Processor  arith_type=Unsigned  bitwidth=32  bin_pt=0  sample_period=1  gw_name=test_loopback_mux_Feng_sim_1_2_3_ip_addr_user_data_out
      link override test_loopback_mux_Feng_sim_1_2_3_ip_addr_user_data_out: arith_type=Unsigned  n_bits=32  bin_pt=0  period=1
  mcnt_cnt : xbsIndex_r4/Counter  cnt_type=Free Running  cnt_to=Inf  operation=Up  start_count=0  cnt_by_val=1  arith_type=Unsigned  n_bits=64  bin_pt=0  load_pin=off  rst=off  en=on  explicit_period=off  period=1  dbl_ovrd=off  use_behavioral_HDL=off  use_rpm=off  implementation=Fabric  block_type=counter
      settings: xl_area=[0, 0, 0, 0, 0, 0, 0]
  negedge : casper_library/Misc/negedge  Tag=Rising Edge Detector  SystemSampleTime=-1
  payload_len : xps_library/software register  Tag=xps:sw_reg  SystemSampleTime=-1  io_dir=From Processor  arith_type=Unsigned  bitwidth=32  bin_pt=0  sample_period=1  gw_name=test_loopback_mux_Feng_sim_1_2_3_payload_len_user_data_out
      link override test_loopback_mux_Feng_sim_1_2_3_payload_len_user_data_out: arith_type=Unsigned  n_bits=32  bin_pt=0  period=1
  period : xps_library/software register  Tag=xps:sw_reg  SystemSampleTime=-1  io_dir=From Processor  arith_type=Unsigned  bitwidth=32  bin_pt=0  sample_period=1  gw_name=test_loopback_mux_Feng_sim_1_2_3_period_user_data_out
      link override test_loopback_mux_Feng_sim_1_2_3_period_user_data_out: arith_type=Unsigned  n_bits=32  bin_pt=0  period=1
  posedge : casper_library/Misc/pulse_ext/posedge  Tag=Rising Edge Detector  SystemSampleTime=-1
  run : xps_library/software register  Tag=xps:sw_reg  SystemSampleTime=-1  io_dir=From Processor  arith_type=Unsigned  bitwidth=32  bin_pt=0  sample_period=1  gw_name=test_loopback_mux_Feng_sim_1_2_3_run_user_data_out
      link override test_loopback_mux_Feng_sim_1_2_3_run_user_data_out: arith_type=Unsigned  n_bits=32  bin_pt=0  period=1
  sim_IP : Constant  OutDataType=sfix(16)  OutScaling=2^0
  sim_freq : Constant  Value=52  OutDataType=sfix(16)  OutScaling=2^0
  sim_length : Constant  Value=50  OutDataType=sfix(16)  OutScaling=2^0
  warn period Convert10 : xbsReplacements_r4/Warning  SystemSampleTime=-1  period=1
  warn period Convert20 : xbsReplacements_r4/Warning  SystemSampleTime=-1  period=1
  warn period Convert30 : xbsReplacements_r4/Warning  SystemSampleTime=-1  period=1
  warn period Relational0 : xbsReplacements_r4/Warning  SystemSampleTime=-1  period=1
  d_out : Outport  OutDataType=sfix(16)  OutScaling=2^0
  valid : Outport  Port=2  OutDataType=sfix(16)  OutScaling=2^0
  dest_ip : Outport  Port=3  OutDataType=sfix(16)  OutScaling=2^0
  eof : Outport  Port=4  OutDataType=sfix(16)  OutScaling=2^0
  discard : Outport  Port=5  OutDataType=sfix(16)  OutScaling=2^0
  wires:
  Counter2/1 -> Relational/1
  Relational/1 -> posedge/1, Counter2/1
  Counter1/1 -> Mux3/3
  negedge/1 -> Convert1/1
  period/1 -> Relational/2
  sim_freq/1 -> period/1
  sim_IP/1 -> ip_addr/1
  Relational5/1 -> Logical/2, Mux2/1, negedge/1, Counter3/2
  Counter3/1 -> Relational5/1, Relational1/2
  posedge/1 -> Counter3/1, Counter4/1, mcnt_cnt/1, Gateway Out1/1
  sim_length/1 -> payload_len/1
  payload_len/1 -> Relational5/2
  Mux/1 -> valid/1, Gateway Out2/1
  Constant/1 -> Mux/2, Mux1/2
  Mux1/1 -> eof/1
  Convert1/1 -> Mux1/3
  Mux3/1 -> d_out/1
  Delay8/1 -> dest_ip/1
  run/1 -> Slice1/1
  Constant2/1 -> run/1
  Slice1/1 -> Mux/1, Mux1/1, Inverter1/1, Convert3/1
  Delay4/1 -> discard/1
  Mux2/1 -> Mux/3
  Inverter/1 -> Counter1/1
  Delay2/1 -> Counter1/2
  Convert3/1 -> Inverter/1
  Constant3/1 -> Mux2/2
  Constant1/1 -> Mux2/3
  Inverter1/1 -> Convert2/1
  Convert2/1 -> Delay4/1
  ip_addr/1 -> Slice/1
  Slice/1 -> AddSub/1
  AddSub/1 -> Delay1/1, Slice2/1
  Constant4/1 -> Relational1/1
  Relational1/1 -> Inverter2/1
  Inverter2/1 -> Delay5/1, Logical/1
  mcnt_cnt/1 -> Slice3/1
  Constant5/1 -> Concat1/2
  Concat1/1 -> Mux3/2, Gateway Out/1
  Delay5/1 -> Mux3/1, Gateway Out4/1
  Gateway Out/1 -> Scope/1
  Gateway Out1/1 -> Scope/2
  Gateway Out2/1 -> Scope/3
  Gateway Out3/1 -> Scope/4
  Gateway Out4/1 -> Scope/5
  Logical/1 -> Delay2/1, Gateway Out3/1
  Slice3/1 -> Concat1/1
  Slice2/1 -> Concat1/3
  Delay1/1 -> Delay8/1
  Counter4/1 -> AddSub/2

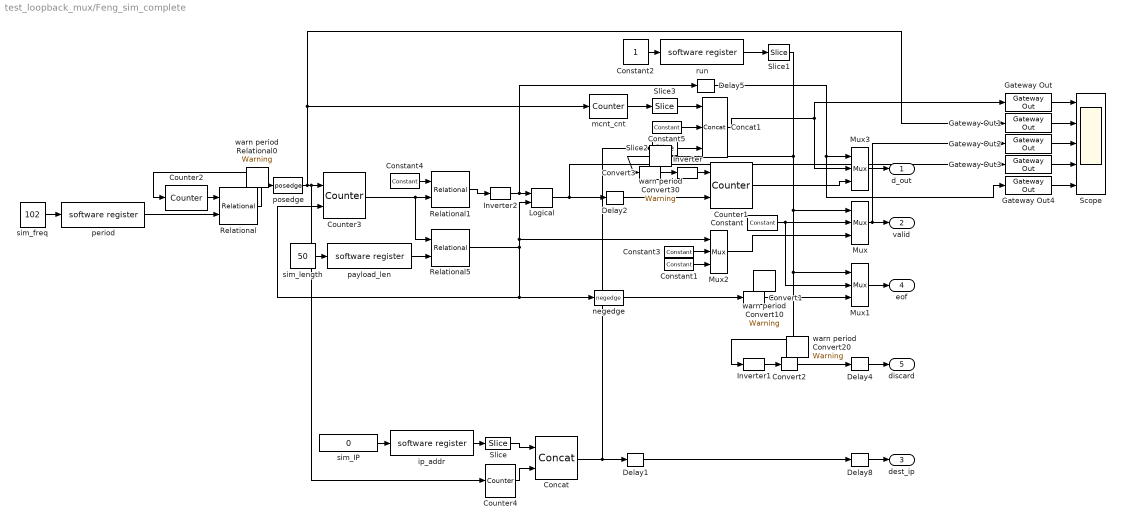
== system test_loopback_mux/Feng_sim_complete ==
  Concat : xbsIndex_r4/Concat  num_inputs=2  dbl_ovrd=off  block_type=concat
      settings: block_version=10.1.3
  Concat1 : xbsIndex_r4/Concat  num_inputs=3  dbl_ovrd=off  block_type=concat
      settings: block_version=10.1.3
  Constant : xbsIndex_r4/Constant  arith_type=Boolean  const=0  n_bits=1  bin_pt=0  explicit_period=on  period=1  equ=P=C  opselect=C  inp2=PCIN>>17  opr=+  inp1=P  carry=CIN  dbl_ovrd=off  block_type=constant
  Constant1 : xbsIndex_r4/Constant  arith_type=Boolean  const=1  n_bits=1  bin_pt=0  explicit_period=off  period=1  equ=P=C  opselect=C  inp2=PCIN>>17  opr=+  inp1=P  carry=CIN  dbl_ovrd=off  block_type=constant
  Constant2 : Constant  OutDataType=sfix(16)  OutScaling=2^0
  Constant3 : xbsIndex_r4/Constant  arith_type=Boolean  const=0  n_bits=1  bin_pt=0  explicit_period=off  period=1  equ=P=C  opselect=C  inp2=PCIN>>17  opr=+  inp1=P  carry=CIN  dbl_ovrd=off  block_type=constant
  Constant4 : xbsIndex_r4/Constant  arith_type=Unsigned  const=0  n_bits=32  bin_pt=0  explicit_period=on  period=1  equ=P=C  opselect=C  inp2=PCIN>>17  opr=+  inp1=P  carry=CIN  dbl_ovrd=off  block_type=constant
  Constant5 : xbsIndex_r4/Constant  arith_type=Unsigned  const=0  n_bits=16-2  bin_pt=0  explicit_period=on  period=1  equ=P=C  opselect=C  inp2=PCIN>>17  opr=+  inp1=P  carry=CIN  dbl_ovrd=off  block_type=constant
  Convert1 : xbsIndex_r4/Convert  arith_type=Boolean  n_bits=8  bin_pt=6  quantization=Truncate  overflow=Wrap  latency=0  dbl_ovrd=off  pipeline=off  block_type=convert
      settings: xl_area=[0, 0, 0, 0, 0, 0, 0]  block_version=10.1.3
  Convert2 : xbsIndex_r4/Convert  arith_type=Boolean  n_bits=8  bin_pt=6  quantization=Truncate  overflow=Wrap  latency=0  dbl_ovrd=off  pipeline=off  block_type=convert
      settings: xl_area=[0, 0, 0, 0, 0, 0, 0]  block_version=10.1.3
  Convert3 : xbsIndex_r4/Convert  arith_type=Boolean  n_bits=8  bin_pt=6  quantization=Truncate  overflow=Wrap  latency=0  dbl_ovrd=off  pipeline=off  block_type=convert
      settings: xl_area=[0, 0, 0, 0, 0, 0, 0]  block_version=10.1.3
  Counter1 : xbsIndex_r4/Counter  cnt_type=Free Running  cnt_to=Inf  operation=Up  start_count=0  cnt_by_val=1  arith_type=Unsigned  n_bits=64  bin_pt=0  load_pin=off  rst=on  en=on  explicit_period=off  period=1  dbl_ovrd=off  use_behavioral_HDL=off  use_rpm=off  implementation=Fabric  block_type=counter
      settings: xl_area=[0, 0, 0, 0, 0, 0, 0]
  Counter2 : xbsIndex_r4/Counter  cnt_type=Free Running  cnt_to=Inf  operation=Up  start_count=1  cnt_by_val=1  arith_type=Unsigned  n_bits=32  bin_pt=0  load_pin=off  rst=on  en=off  explicit_period=on  period=1  dbl_ovrd=off  use_behavioral_HDL=off  use_rpm=on  implementation=Fabric  block_type=counter
      settings: xl_area=[0, 0, 0, 0, 0, 0, 0]
  Counter3 : xbsIndex_r4/Counter  cnt_type=Free Running  cnt_to=1023  operation=Up  start_count=0  cnt_by_val=1  arith_type=Unsigned  n_bits=32  bin_pt=0  load_pin=off  rst=on  en=on  explicit_period=on  period=1  dbl_ovrd=off  use_behavioral_HDL=off  use_rpm=on  implementation=Fabric  block_type=counter
      settings: xl_area=[0, 0, 0, 0, 0, 0, 0]
  Counter4 : xbsIndex_r4/Counter  cnt_type=Free Running  cnt_to=1023  operation=Up  start_count=0  cnt_by_val=1  arith_type=Unsigned  n_bits=2  bin_pt=0  load_pin=off  rst=off  en=on  explicit_period=on  period=1  dbl_ovrd=off  use_behavioral_HDL=off  use_rpm=on  implementation=Fabric  block_type=counter
      settings: xl_area=[0, 0, 0, 0, 0, 0, 0]
  Delay{1..2,4..5,8} (5 alike) : xbsIndex_r4/Delay  en=off  latency=1  dbl_ovrd=off  reg_retiming=on  block_type=delay
      settings: xl_area=[0, 0, 0, 0, 0, 0, 0]
  Gateway Out{,1..4} (5 alike) : xbsIndex_r4/Gateway Out  hdl_port=on  timing_constraint=None  locs_specified=off  LOCs={}  block_type=gatewayout
      settings: infoedit="Gateway out block.  Converts Xilinx fixed point inputs into ouputs of type Simulink integer, double, or fixed point.<P><P>Hardware notes:  In hardware these blocks become top level output ports or are discarded, depending on how they are configured."  xl_area=[0, 0, 0, 0, 0, 0, 0]  block_version=10.1.3
  Inverter : xbsIndex_r4/Inverter  en=off  latency=0  dbl_ovrd=off  block_type=inv
      settings: xl_area=[0, 0, 0, 0, 0, 0, 0]
  Inverter1 : xbsIndex_r4/Inverter  en=off  latency=0  dbl_ovrd=off  block_type=inv
      settings: xl_area=[0, 0, 0, 0, 0, 0, 0]
  Inverter2 : xbsIndex_r4/Inverter  en=off  latency=0  dbl_ovrd=off  block_type=inv
      settings: xl_area=[0, 0, 0, 0, 0, 0, 0]
  Logical : xbsIndex_r4/Logical  logical_function=AND  inputs=2  en=off  latency=0  precision=Full  arith_type=Unsigned  n_bits=8  bin_pt=2  align_bp=on  dbl_ovrd=off  block_type=logical
      settings: xl_area=[0, 0, 0, 0, 0, 0, 0]
  Mux{,1..3} (4 alike) : xbsIndex_r4/Mux  inputs=2  en=off  latency=1  precision=Full  arith_type="Signed  (2's comp)"  n_bits=8  bin_pt=2  quantization=Truncate  overflow=Wrap  dbl_ovrd=off  block_type=mux
      settings: xl_area=[0, 0, 0, 0, 0, 0, 0]
  Relational : xbsIndex_r4/Relational  mode=a>=b  en=off  latency=0  dbl_ovrd=off  block_type=relational
      settings: xl_area=[0, 0, 0, 0, 0, 0, 0]  block_version=10.1.3
  Relational1 : xbsIndex_r4/Relational  mode=a=b  en=off  latency=0  dbl_ovrd=off  block_type=relational
      settings: xl_area=[0, 0, 0, 0, 0, 0, 0]  block_version=10.1.3
  Relational5 : xbsIndex_r4/Relational  mode=a<=b  en=off  latency=0  dbl_ovrd=off  block_type=relational
      settings: xl_area=[0, 0, 0, 0, 0, 0, 0]  block_version=10.1.3
  Scope : Scope  NumInputPorts=5
      settings: TimeRange=4000  YMin=130000~0~0~0~0  YMax=200000~1~1~1~1  SaveName=ScopeData11
  Slice : xbsIndex_r4/Slice  nbits=30  boolean_output=off  mode=Upper Bit Location + Width  bit1=0  base1=MSB of Input  bit0=0  base0=LSB of Input  dbl_ovrd=off  block_type=slice
      settings: infoedit="Extracts a given range of bits from each input sample and presents it at the output.  The output type is ordinarily unsigned with binary point at zero, but can be Boolean when the slice is one bit wide.<P><P>Hardware notes: In hardware this block costs nothing."  block_version=10.1.3
  Slice1 : xbsIndex_r4/Slice  nbits=1  boolean_output=off  mode=Lower Bit Location + Width  bit1=1  base1=MSB of Input  bit0=0  base0=LSB of Input  dbl_ovrd=off  block_type=slice
      settings: infoedit="Extracts a given range of bits from each input sample and presents it at the output.  The output type is ordinarily unsigned with binary point at zero, but can be Boolean when the slice is one bit wide.<P><P>Hardware notes: In hardware this block costs nothing."  block_version=10.1.3
  Slice2 : xbsIndex_r4/Slice  nbits=2  boolean_output=off  mode=Lower Bit Location + Width  bit1=1  base1=MSB of Input  bit0=0  base0=LSB of Input  dbl_ovrd=off  block_type=slice
      settings: infoedit="Extracts a given range of bits from each input sample and presents it at the output.  The output type is ordinarily unsigned with binary point at zero, but can be Boolean when the slice is one bit wide.<P><P>Hardware notes: In hardware this block costs nothing."  block_version=10.1.3
  Slice3 : xbsIndex_r4/Slice  nbits=48  boolean_output=off  mode=Lower Bit Location + Width  bit1=1  base1=MSB of Input  bit0=3  base0=LSB of Input  dbl_ovrd=off  block_type=slice
      settings: infoedit="Extracts a given range of bits from each input sample and presents it at the output.  The output type is ordinarily unsigned with binary point at zero, but can be Boolean when the slice is one bit wide.<P><P>Hardware notes: In hardware this block costs nothing."  block_version=10.1.3
  ip_addr : xps_library/software register  Tag=xps:sw_reg  SystemSampleTime=-1  io_dir=From Processor  arith_type=Unsigned  bitwidth=32  bin_pt=0  sample_period=1  gw_name=test_loopback_mux_Feng_sim_complete_ip_addr_user_data_out
      link override test_loopback_mux_Feng_sim_complete_ip_addr_user_data_out: arith_type=Unsigned  n_bits=32  bin_pt=0  period=1
  mcnt_cnt : xbsIndex_r4/Counter  cnt_type=Free Running  cnt_to=Inf  operation=Up  start_count=0  cnt_by_val=1  arith_type=Unsigned  n_bits=64  bin_pt=0  load_pin=off  rst=off  en=on  explicit_period=off  period=1  dbl_ovrd=off  use_behavioral_HDL=off  use_rpm=off  implementation=Fabric  block_type=counter
      settings: xl_area=[0, 0, 0, 0, 0, 0, 0]
  negedge : casper_library/Misc/negedge  Tag=Rising Edge Detector  SystemSampleTime=-1
  payload_len : xps_library/software register  Tag=xps:sw_reg  SystemSampleTime=-1  io_dir=From Processor  arith_type=Unsigned  bitwidth=32  bin_pt=0  sample_period=1  gw_name=test_loopback_mux_Feng_sim_complete_payload_len_user_data_out
      link override test_loopback_mux_Feng_sim_complete_payload_len_user_data_out: arith_type=Unsigned  n_bits=32  bin_pt=0  period=1
  period : xps_library/software register  Tag=xps:sw_reg  SystemSampleTime=-1  io_dir=From Processor  arith_type=Unsigned  bitwidth=32  bin_pt=0  sample_period=1  gw_name=test_loopback_mux_Feng_sim_complete_period_user_data_out
      link override test_loopback_mux_Feng_sim_complete_period_user_data_out: arith_type=Unsigned  n_bits=32  bin_pt=0  period=1
  posedge : casper_library/Misc/pulse_ext/posedge  Tag=Rising Edge Detector  SystemSampleTime=-1
  run : xps_library/software register  Tag=xps:sw_reg  SystemSampleTime=-1  io_dir=From Processor  arith_type=Unsigned  bitwidth=32  bin_pt=0  sample_period=1  gw_name=test_loopback_mux_Feng_sim_complete_run_user_data_out
      link override test_loopback_mux_Feng_sim_complete_run_user_data_out: arith_type=Unsigned  n_bits=32  bin_pt=0  period=1
  sim_IP : Constant  Value=0  OutDataType=sfix(16)  OutScaling=2^0
  sim_freq : Constant  Value=102  OutDataType=sfix(16)  OutScaling=2^0
  sim_length : Constant  Value=50  OutDataType=sfix(16)  OutScaling=2^0
  warn period Convert10 : xbsReplacements_r4/Warning  SystemSampleTime=-1  period=1
  warn period Convert20 : xbsReplacements_r4/Warning  SystemSampleTime=-1  period=1
  warn period Convert30 : xbsReplacements_r4/Warning  SystemSampleTime=-1  period=1
  warn period Relational0 : xbsReplacements_r4/Warning  SystemSampleTime=-1  period=1
  d_out : Outport  OutDataType=sfix(16)  OutScaling=2^0
  valid : Outport  Port=2  OutDataType=sfix(16)  OutScaling=2^0
  dest_ip : Outport  Port=3  OutDataType=sfix(16)  OutScaling=2^0
  eof : Outport  Port=4  OutDataType=sfix(16)  OutScaling=2^0
  discard : Outport  Port=5  OutDataType=sfix(16)  OutScaling=2^0
  wires:
  Counter2/1 -> Relational/1
  Relational/1 -> posedge/1, Counter2/1
  Counter1/1 -> Mux3/3
  negedge/1 -> Convert1/1
  period/1 -> Relational/2
  sim_freq/1 -> period/1
  sim_IP/1 -> ip_addr/1
  Relational5/1 -> Logical/2, Mux2/1, negedge/1, Counter3/2
  Counter3/1 -> Relational5/1, Relational1/2
  posedge/1 -> Counter3/1, Counter4/1, mcnt_cnt/1, Gateway Out1/1
  sim_length/1 -> payload_len/1
  payload_len/1 -> Relational5/2
  Mux/1 -> valid/1, Gateway Out2/1
  Constant/1 -> Mux/2, Mux1/2
  Mux1/1 -> eof/1
  Convert1/1 -> Mux1/3
  Mux3/1 -> d_out/1
  Delay8/1 -> dest_ip/1
  run/1 -> Slice1/1
  Constant2/1 -> run/1
  Slice1/1 -> Mux/1, Mux1/1, Inverter1/1, Convert3/1
  Delay4/1 -> discard/1
  Mux2/1 -> Mux/3
  Inverter/1 -> Counter1/1
  Delay2/1 -> Counter1/2
  Convert3/1 -> Inverter/1
  Constant3/1 -> Mux2/2
  Constant1/1 -> Mux2/3
  Inverter1/1 -> Convert2/1
  Convert2/1 -> Delay4/1
  ip_addr/1 -> Slice/1
  Counter4/1 -> Concat/2
  Slice/1 -> Concat/1
  Concat/1 -> Delay1/1, Slice2/1
  Constant4/1 -> Relational1/1
  Relational1/1 -> Inverter2/1
  Inverter2/1 -> Delay5/1, Logical/1
  mcnt_cnt/1 -> Slice3/1
  Constant5/1 -> Concat1/2
  Concat1/1 -> Mux3/2, Gateway Out/1
  Delay5/1 -> Mux3/1, Gateway Out4/1
  Gateway Out/1 -> Scope/1
  Gateway Out1/1 -> Scope/2
  Gateway Out2/1 -> Scope/3
  Gateway Out3/1 -> Scope/4
  Gateway Out4/1 -> Scope/5
  Logical/1 -> Delay2/1, Gateway Out3/1
  Slice3/1 -> Concat1/1
  Slice2/1 -> Concat1/3
  Delay1/1 -> Delay8/1
